simulink model "Kalman_Filter_Onde_Dim"  (Simulink 6.6)
settings: Solver=VariableStepDiscrete  StartTime=0.0  StopTime=10.0  RelTol=1e-3
libraries: dspsrcs4 x2, simulink x1, dspadpt3 x1
settings Model: Creator=LIGHT  LastModifiedBy=light
settings DataIOCC: MaxDataPoints=2000

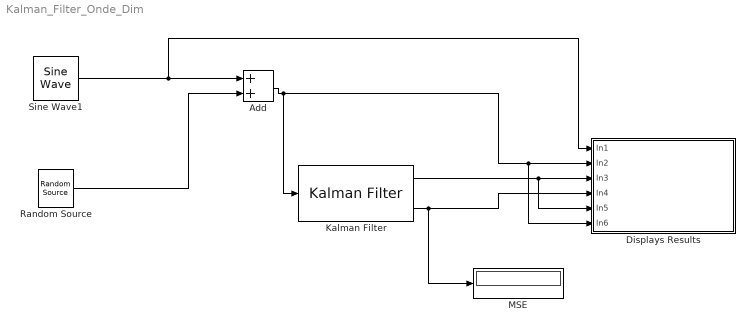
== system Kalman_Filter_Onde_Dim ==
  Add : Sum  OutDataTypeMode=double  OutScaling=2^-10  RndMeth=Nearest  SampleTime=1/1000  InputSameDT=on
  Displays Results : Subsystem
  Kalman Filter : dspadpt3/Kalman Filter  DialogController=dspDDGCreate  DialogControllerArgs=DataTag0  SystemSampleTime=-1  num_targets=1  sourceEnable=Always  isReset=on  X=1.00  P=0.90  A=1.00  sourceMeasure=Specify via Dialog  H=1.00  Q=0.01  R=2  isOutputEstMeasure=off  isOutputEstState=on  isOutputEstError=on  isOutputPrdMeasure=off  isOutputPrdState=off  isOutputPrdError=off
  MSE : Display
  Random Source : dspsrcs4/Random Source  SrcType=Gaussian  NormMethod=Ziggurat  CltLength=12  MinVal=0  MaxVal=1  MeanVal=0  VarVal=1  RepMode=Not repeatable  rawSeed=1  IsInherit=off  SampMode=Discrete  SampTime=1/1000  SampFrame=1  DataType=Double  OutComplex=Real
  Sine Wave1 : dspsrcs4/Sine Wave  Amplitude=3  Frequency=2  Phase=0  SampleMode=Discrete  OutComplex=Real  CompMethod=Trigonometric fcn  TableSize=Speed  SampleTime=1/1000  SamplesPerFrame=1  dataType=double  wordLen=16  udDataType=sfix(16)  fracBitsMode=Best precision  numFracBits=15  ResetState=Catch up to simulation time
  wires:
  Add/1 -> Kalman Filter/1, Displays Results/2(In2), Displays Results/6(In6)
  Sine Wave1/1 -> Add/1, Displays Results/1(In1)
  Random Source/1 -> Add/2
  Kalman Filter/2 -> Displays Results/4(In4), MSE/1
  Kalman Filter/1 -> Displays Results/3(In3), Displays Results/5(In5)

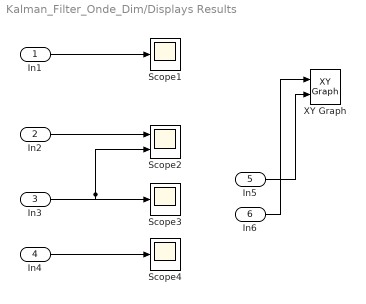
== system Kalman_Filter_Onde_Dim/Displays Results ==
  In1 : Inport
  In2 : Inport  Port=2
  In3 : Inport  Port=3
  In4 : Inport  Port=4
  In5 : Inport  Port=5
  In6 : Inport  Port=6
  Scope1 : Scope
      settings: Tag=Original Sine Wave  Priority=1  AttributesFormatString=Original signal  TimeRange=10
  Scope2 : Scope  NumInputPorts=2
      settings: TimeRange=5  YMin=-6~-5  YMax=6~5
  Scope3 : Scope
      settings: SaveName=ScopeData2
  Scope4 : Scope
      settings: SaveName=ScopeData3
  XY Graph : simulink/Sinks/XY Graph  SystemSampleTime=-1  xmin=-10  xmax=10  ymin=-10  ymax=10  st=1/1000
  wires:
  In1/1 -> Scope1/1
  In2/1 -> Scope2/1
  In4/1 -> Scope4/1
  In6/1 -> XY Graph/1
  In5/1 -> XY Graph/2
  In3/1 -> Scope2/2, Scope3/1
